simulink model "SA_3pannels_aug"  (R2025b)
settings: Solver=VariableStepAuto  StartTime=0.0  StopTime=10.0  RelTol=1e-3
libraries: RCTblocks x3
settings Model: Creator=d.alazard  LastModifiedBy=andre
settings SolverCC: AlgebraicLoopSolver=TrustRegion
settings DataIOCC: ReturnWorkspaceOutputs=off
settings DebuggingCC: AlgebraicLoopMsg=none  UnconnectedInputMsg=warning  UnconnectedOutputMsg=warning  UnconnectedLineMsg=warning  ArithmeticOperatorsInVariantConditions=warning
settings ModelReferenceCC: EnableRefExpFcnMdlSchedulingChecks=on
settings SFSimCC: CustomCodeUndefinedFunction=UseInterfaceOnly
settings RTWCC: GPUComputeCapability=3.5  DLArmComputeVersion=19.05

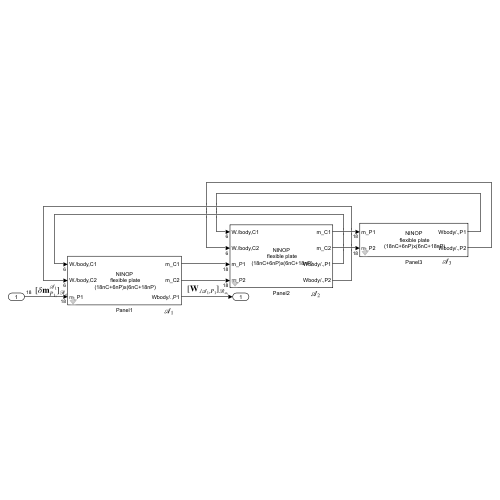
[thumbnail: Simulink's stored preview of the top-level diagram]
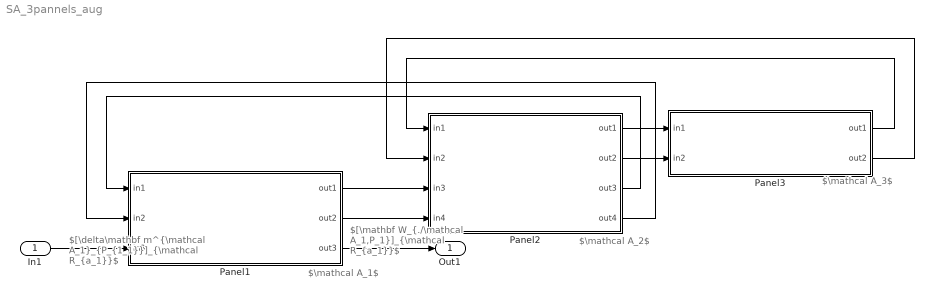
== system SA_3pannels_aug ==
  note: $[\mathbf W_{./\mathcal A_1,P_1}]_{\mathcal R_{a_1}}$
  note: $[\delta\mathbf m^{\mathcal A_1}_{P_{1_1}}]_{\mathcal R_{a_1}}$
  note: $\mathcal A_1$
  note: $\mathcal A_2$
  note: $\mathcal A_3$
  In1 : Inport  PortDimensions=18
  Panel1 : Subsystem  mask(Multi-port flexible plate (18nC+6nP)x(6nC+18nP)){lx=1, ly=1, t=0.01, rho=474, E=44e9, ni=0.35, xi=0.005, i_nP=1, i_nC=2, OP1=[0;0.5;0], OP2=[1;1;0], OP3=[1;0;0], OP4=[1;1;0], OC1=[1;0.75;0], OC2=[1;0.25;0], OC3=[1;0;0], OC4=[1;1;0], OC5=[1;1;0], OC6=[0;1;0], OC7=[0;0;0], OC8=[0;0;0], RedSlowOn=off, uw_var=0, Nflex=0}
      mask prompts: lx "lenght along x (m)"; ly "length along y (m)"; t "thickness (m)"; rho "Mass density (Kg/m^3)"; E "Young modulus (N/m^2)"; ni "Poisson coefficient"; xi "damping coefficient"; i_nP "Number of parent (P) nodes (<5)"; i_nC "Number of child (C) nodes"; OP1 "OP1 (3x1 vector: [x;y;0], m)"; OP2 "OP2 (3x1 vectorr: [x;y;0], m)"; OP3 "OP3 (3x1 vectorr: [x;y;0], m)"; OP4 "OP4 (3x1 vectorr: [x;y;0], m)"; OC1 "OC1 (3x1 vectorr: [x;y;0], m)"; OC2 "OC2 (3x1 vectorr: [x;y;0], m)"; OC3 "OC3 (3x1 vectorr: [x;y;0], m)"; OC4 "OC4 (3x1 vectorr: [x;y;0], m)"; OC5 "OC5 (3x1 vectorr: [x;y;0], m)"; OC6 "OC6 (3x1 vectorr: [x;y;0], m)"; OC7 "OC7 (3x1 vector: [x;y;0],m)"; OC8 "OC8 (3x1 vector [x;y;0], m)"; RedSlowOn "Reduction of the 6*(nP-1) poles at 0 (due to loop closure constraints when nP>1)."; uw_var "uncertainty (%)"; Nflex "number of flexible modes (Nf, integer)"
      mask help:
      | (18nC+6nP)x(6nC+18nP) multi-port model of a uniform plate (in the x-y plane) between
      |   *  wrenches applied to the plate at the given nC child nodes (input) and motion vectors at these child nodes (output)
      |   *  motion vectors at the nP parent nodes (input)  and wrenches applied by this plate at these parent nodes (output)
      |  dynamic model of a uniform flexible plate (in the x-y plane),
      | in the plate reference frame (0,x,y,z)
      |
      | The plate is defined by:
      | * 0<x<lx
      | * 0<y<ly
      | * -t/2<z<t/2
      |
      | All parameters are expressed in the plate reference frame.
      | Dynamics in translations along x and y and rotation around z are assumed rigid.
      mask init:
      | MultiPortFlexiblePlateAug
      mask Help: web('DocPlate_joly.html','-browser')
      mask TypeOptions i_nP: 0 | 1 | 2 | 3 | 4
      mask TypeOptions i_nC: 0 | 1 | 2 | 3 | 4 | 5 | 6 | 7 | 8
      mask DialogControl ParameterGroupVar Prompt: Main parameters
      mask DialogControl Pport1 Prompt: P node #1
      mask DialogControl Pport2 Prompt: #2
      mask DialogControl Pport3 Prompt: #3
      mask DialogControl Pport4 Prompt: #4
      mask DialogControl Cport1 Prompt: C node #1
      mask DialogControl Cport2 Prompt: #2
      mask DialogControl Cport3 Prompt: #3
      mask DialogControl Cport4 Prompt: #4
      mask DialogControl Cport5 Prompt: #5
      mask DialogControl Cport6 Prompt: #6
      mask DialogControl Cport7 Prompt: #7
      mask DialogControl Cport8 Prompt: #8
      mask DialogControl Reduction Prompt: Optional Reduction
      mask DialogControl Container19 Prompt: Parametric uncertainties
      mask DialogControl Control8 Prompt: The uncertain parameters are the first Nf cantilevered frequencies of the plate when it is clamped at the first parent node (P1) or the last child node when the number of parent nodes is null.
      mask DialogControl Control4 Prompt: The uncertain frequency is named: 'w_name_i' where:
      mask DialogControl Control5 Prompt: * 'name' is the current block name (reduced to its alphanumeric characters).
      mask DialogControl Control6 Prompt: * 'i' is the flexible mode number (increasing frequency order)
      mask Display:
      | disp('NINOP\n flexible plate\n (18nC+6nP)x(6nC+18nP)')
      | if nC~=0
      |     for ii=1:nC
      |         port_label('input', ii, ['W./body,C',num2str(ii)])
      |         port_label('output',ii,['m_C',num2str(ii)])
      |     end
      | end
      | if nP~=0
      |     for ii=1:nP
      |         port_label('input', nC+ii, ['m_P',num2str(ii)])
      |         port_label('output',nC+ii,['Wbody/.,P',num2str(ii)])
      |     end
      | end
  Panel2 : Subsystem  mask(Multi-port flexible plate (18nC+6nP)x(6nC+18nP)){lx=1, ly=1, t=0.01, rho=474, E=44e9, ni=0.35, xi=0.005, i_nP=2, i_nC=2, OP1=[0;0.75;0], OP2=[0;0.25;0], OP3=[1;0;0], OP4=[1;1;0], OC1=[1;0.75;0], OC2=[1;0.25;0], OC3=[1;0;0], OC4=[1;1;0], OC5=[1;1;0], OC6=[0;1;0], OC7=[0;0;0], OC8=[0;0;0], RedSlowOn=off, uw_var=0, Nflex=0}
      mask prompts: lx "lenght along x (m)"; ly "length along y (m)"; t "thickness (m)"; rho "Mass density (Kg/m^3)"; E "Young modulus (N/m^2)"; ni "Poisson coefficient"; xi "damping coefficient"; i_nP "Number of parent (P) nodes (<5)"; i_nC "Number of child (C) nodes"; OP1 "OP1 (3x1 vector: [x;y;0], m)"; OP2 "OP2 (3x1 vectorr: [x;y;0], m)"; OP3 "OP3 (3x1 vectorr: [x;y;0], m)"; OP4 "OP4 (3x1 vectorr: [x;y;0], m)"; OC1 "OC1 (3x1 vectorr: [x;y;0], m)"; OC2 "OC2 (3x1 vectorr: [x;y;0], m)"; OC3 "OC3 (3x1 vectorr: [x;y;0], m)"; OC4 "OC4 (3x1 vectorr: [x;y;0], m)"; OC5 "OC5 (3x1 vectorr: [x;y;0], m)"; OC6 "OC6 (3x1 vectorr: [x;y;0], m)"; OC7 "OC7 (3x1 vector: [x;y;0],m)"; OC8 "OC8 (3x1 vector [x;y;0], m)"; RedSlowOn "Reduction of the 6*(nP-1) poles at 0 (due to loop closure constraints when nP>1)."; uw_var "uncertainty (%)"; Nflex "number of flexible modes (Nf, integer)"
      mask help:
      | (18nC+6nP)x(6nC+18nP) multi-port model of a uniform plate (in the x-y plane) between
      |   *  wrenches applied to the plate at the given nC child nodes (input) and motion vectors at these child nodes (output)
      |   *  motion vectors at the nP parent nodes (input)  and wrenches applied by this plate at these parent nodes (output)
      |  dynamic model of a uniform flexible plate (in the x-y plane),
      | in the plate reference frame (0,x,y,z)
      |
      | The plate is defined by:
      | * 0<x<lx
      | * 0<y<ly
      | * -t/2<z<t/2
      |
      | All parameters are expressed in the plate reference frame.
      | Dynamics in translations along x and y and rotation around z are assumed rigid.
      mask init:
      | MultiPortFlexiblePlateAug
      mask Help: web('DocPlate_joly.html','-browser')
      mask TypeOptions i_nP: 0 | 1 | 2 | 3 | 4
      mask TypeOptions i_nC: 0 | 1 | 2 | 3 | 4 | 5 | 6 | 7 | 8
      mask DialogControl ParameterGroupVar Prompt: Main parameters
      mask DialogControl Pport1 Prompt: P node #1
      mask DialogControl Pport2 Prompt: #2
      mask DialogControl Pport3 Prompt: #3
      mask DialogControl Pport4 Prompt: #4
      mask DialogControl Cport1 Prompt: C node #1
      mask DialogControl Cport2 Prompt: #2
      mask DialogControl Cport3 Prompt: #3
      mask DialogControl Cport4 Prompt: #4
      mask DialogControl Cport5 Prompt: #5
      mask DialogControl Cport6 Prompt: #6
      mask DialogControl Cport7 Prompt: #7
      mask DialogControl Cport8 Prompt: #8
      mask DialogControl Reduction Prompt: Optional Reduction
      mask DialogControl Container19 Prompt: Parametric uncertainties
      mask DialogControl Control8 Prompt: The uncertain parameters are the first Nf cantilevered frequencies of the plate when it is clamped at the first parent node (P1) or the last child node when the number of parent nodes is null.
      mask DialogControl Control4 Prompt: The uncertain frequency is named: 'w_name_i' where:
      mask DialogControl Control5 Prompt: * 'name' is the current block name (reduced to its alphanumeric characters).
      mask DialogControl Control6 Prompt: * 'i' is the flexible mode number (increasing frequency order)
      mask Display:
      | disp('NINOP\n flexible plate\n (18nC+6nP)x(6nC+18nP)')
      | if nC~=0
      |     for ii=1:nC
      |         port_label('input', ii, ['W./body,C',num2str(ii)])
      |         port_label('output',ii,['m_C',num2str(ii)])
      |     end
      | end
      | if nP~=0
      |     for ii=1:nP
      |         port_label('input', nC+ii, ['m_P',num2str(ii)])
      |         port_label('output',nC+ii,['Wbody/.,P',num2str(ii)])
      |     end
      | end
  Panel3 : Subsystem  mask(Multi-port flexible plate (18nC+6nP)x(6nC+18nP)){lx=1, ly=1, t=0.01, rho=474, E=44e9, ni=0.35, xi=0.005, i_nP=2, i_nC=0, OP1=[0;0.75;0], OP2=[0;0.25;0], OP3=[1;0;0], OP4=[1;1;0], OC1=[1;0.75;0], OC2=[1;0.25;0], OC3=[1;0;0], OC4=[1;1;0], OC5=[1;1;0], OC6=[0;1;0], OC7=[0;0;0], OC8=[0;0;0], RedSlowOn=off, uw_var=0, Nflex=0}
      mask prompts: lx "lenght along x (m)"; ly "length along y (m)"; t "thickness (m)"; rho "Mass density (Kg/m^3)"; E "Young modulus (N/m^2)"; ni "Poisson coefficient"; xi "damping coefficient"; i_nP "Number of parent (P) nodes (<5)"; i_nC "Number of child (C) nodes"; OP1 "OP1 (3x1 vector: [x;y;0], m)"; OP2 "OP2 (3x1 vectorr: [x;y;0], m)"; OP3 "OP3 (3x1 vectorr: [x;y;0], m)"; OP4 "OP4 (3x1 vectorr: [x;y;0], m)"; OC1 "OC1 (3x1 vectorr: [x;y;0], m)"; OC2 "OC2 (3x1 vectorr: [x;y;0], m)"; OC3 "OC3 (3x1 vectorr: [x;y;0], m)"; OC4 "OC4 (3x1 vectorr: [x;y;0], m)"; OC5 "OC5 (3x1 vectorr: [x;y;0], m)"; OC6 "OC6 (3x1 vectorr: [x;y;0], m)"; OC7 "OC7 (3x1 vector: [x;y;0],m)"; OC8 "OC8 (3x1 vector [x;y;0], m)"; RedSlowOn "Reduction of the 6*(nP-1) poles at 0 (due to loop closure constraints when nP>1)."; uw_var "uncertainty (%)"; Nflex "number of flexible modes (Nf, integer)"
      mask help:
      | (18nC+6nP)x(6nC+18nP) multi-port model of a uniform plate (in the x-y plane) between
      |   *  wrenches applied to the plate at the given nC child nodes (input) and motion vectors at these child nodes (output)
      |   *  motion vectors at the nP parent nodes (input)  and wrenches applied by this plate at these parent nodes (output)
      |  dynamic model of a uniform flexible plate (in the x-y plane),
      | in the plate reference frame (0,x,y,z)
      |
      | The plate is defined by:
      | * 0<x<lx
      | * 0<y<ly
      | * -t/2<z<t/2
      |
      | All parameters are expressed in the plate reference frame.
      | Dynamics in translations along x and y and rotation around z are assumed rigid.
      mask init:
      | MultiPortFlexiblePlateAug
      mask Help: web('DocPlate_joly.html','-browser')
      mask TypeOptions i_nP: 0 | 1 | 2 | 3 | 4
      mask TypeOptions i_nC: 0 | 1 | 2 | 3 | 4 | 5 | 6 | 7 | 8
      mask DialogControl ParameterGroupVar Prompt: Main parameters
      mask DialogControl Pport1 Prompt: P node #1
      mask DialogControl Pport2 Prompt: #2
      mask DialogControl Pport3 Prompt: #3
      mask DialogControl Pport4 Prompt: #4
      mask DialogControl Cport1 Prompt: C node #1
      mask DialogControl Cport2 Prompt: #2
      mask DialogControl Cport3 Prompt: #3
      mask DialogControl Cport4 Prompt: #4
      mask DialogControl Cport5 Prompt: #5
      mask DialogControl Cport6 Prompt: #6
      mask DialogControl Cport7 Prompt: #7
      mask DialogControl Cport8 Prompt: #8
      mask DialogControl Reduction Prompt: Optional Reduction
      mask DialogControl Container19 Prompt: Parametric uncertainties
      mask DialogControl Control8 Prompt: The uncertain parameters are the first Nf cantilevered frequencies of the plate when it is clamped at the first parent node (P1) or the last child node when the number of parent nodes is null.
      mask DialogControl Control4 Prompt: The uncertain frequency is named: 'w_name_i' where:
      mask DialogControl Control5 Prompt: * 'name' is the current block name (reduced to its alphanumeric characters).
      mask DialogControl Control6 Prompt: * 'i' is the flexible mode number (increasing frequency order)
      mask Display:
      | disp('NINOP\n flexible plate\n (18nC+6nP)x(6nC+18nP)')
      | if nC~=0
      |     for ii=1:nC
      |         port_label('input', ii, ['W./body,C',num2str(ii)])
      |         port_label('output',ii,['m_C',num2str(ii)])
      |     end
      | end
      | if nP~=0
      |     for ii=1:nP
      |         port_label('input', nC+ii, ['m_P',num2str(ii)])
      |         port_label('output',nC+ii,['Wbody/.,P',num2str(ii)])
      |     end
      | end
  Out1 : Outport  VectorParamsAs1DForOutWhenUnconnected=off
  wires:
  In1/1 -> Panel1/3(in3)
  Panel1/3(out3) -> Out1/1
  Panel1/1(out1) -> Panel2/3(in3)
  Panel1/2(out2) -> Panel2/4(in4)
  Panel2/4(out4) -> Panel1/2(in2)
  Panel2/3(out3) -> Panel1/1(in1)
  Panel2/1(out1) -> Panel3/1(in1)
  Panel2/2(out2) -> Panel3/2(in2)
  Panel3/1(out1) -> Panel2/1(in1)
  Panel3/2(out2) -> Panel2/2(in2)

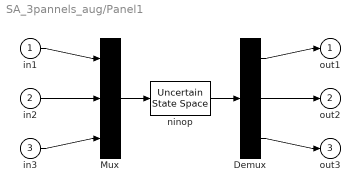
== system SA_3pannels_aug/Panel1 ==
  in1 : Inport  PortDimensions=6
  in2 : Inport  Port=2  PortDimensions=6
  in3 : Inport  Port=3  PortDimensions=18
  Demux : Demux  Outputs=[18 18 6 ]
  Mux : Mux  Inputs=[6 6 18 ]
  ninop : RCTblocks/Uncertain State Space  Tag=USS  USystem=NINOP  UValue=[]  X0=[]  uX0=[]
  out1 : Outport
  out2 : Outport  Port=2
  out3 : Outport  Port=3
  wires:
  Mux/1 -> ninop/1
  ninop/1 -> Demux/1
  in1/1 -> Mux/1
  Demux/1 -> out1/1
  in2/1 -> Mux/2
  Demux/2 -> out2/1
  in3/1 -> Mux/3
  Demux/3 -> out3/1

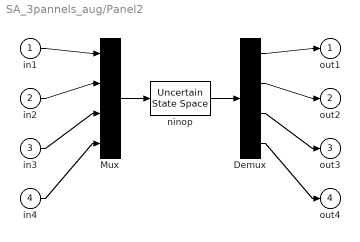
== system SA_3pannels_aug/Panel2 ==
  in1 : Inport  PortDimensions=6
  in2 : Inport  Port=2  PortDimensions=6
  in3 : Inport  Port=3  PortDimensions=18
  in4 : Inport  Port=4  PortDimensions=18
  Demux : Demux  Outputs=[18 18 6 6 ]
  Mux : Mux  Inputs=[6 6 18 18 ]
  ninop : RCTblocks/Uncertain State Space  Tag=USS  USystem=NINOP  UValue=[]  X0=[]  uX0=[]
  out1 : Outport
  out2 : Outport  Port=2
  out3 : Outport  Port=3
  out4 : Outport  Port=4
  wires:
  Mux/1 -> ninop/1
  ninop/1 -> Demux/1
  in1/1 -> Mux/1
  Demux/1 -> out1/1
  in2/1 -> Mux/2
  Demux/2 -> out2/1
  in3/1 -> Mux/3
  Demux/3 -> out3/1
  in4/1 -> Mux/4
  Demux/4 -> out4/1

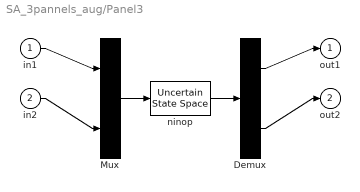
== system SA_3pannels_aug/Panel3 ==
  in1 : Inport  PortDimensions=18
  in2 : Inport  Port=2  PortDimensions=18
  Demux : Demux  Outputs=[6 6 ]
  Mux : Mux  Inputs=[18 18 ]
  ninop : RCTblocks/Uncertain State Space  Tag=USS  USystem=NINOP  UValue=[]  X0=[]  uX0=[]
  out1 : Outport
  out2 : Outport  Port=2
  wires:
  Mux/1 -> ninop/1
  ninop/1 -> Demux/1
  in1/1 -> Mux/1
  Demux/1 -> out1/1
  in2/1 -> Mux/2
  Demux/2 -> out2/1
